simulink model "lab07_Arduino"  (R2022b)
settings: Solver=FixedStepAuto  StartTime=0.0  StopTime=inf  RelTol=1e-3
libraries: arduinolib x4, simulink x3
(part 2 of 2)

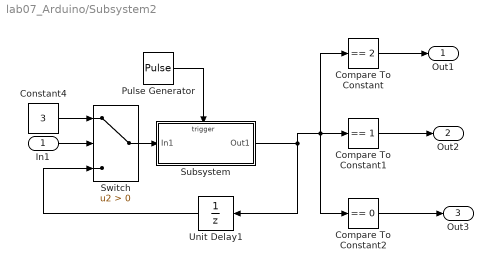
== system lab07_Arduino/Subsystem2 ==
  In1 : Inport
  Compare To Constant : simulink/Logic and Bit Operations/Compare To Constant  relop===  const=2  OutDataTypeStr=boolean
  Compare To Constant1 : simulink/Logic and Bit Operations/Compare To Constant  relop===  const=1  OutDataTypeStr=boolean
  Compare To Constant2 : simulink/Logic and Bit Operations/Compare To Constant  relop===  const=0  OutDataTypeStr=boolean
  Constant4 : Constant  Value=3
  Pulse Generator : DiscretePulseGenerator  PulseType=Time based  Period=5
  Subsystem : Subsystem
  Switch : Switch  Criteria=u2 > Threshold  SaturateOnIntegerOverflow=off  InputSameDT=off
  Unit Delay1 : UnitDelay  SampleTime=-1  HasFrameUpgradeWarning=on
  Out1 : Outport
  Out2 : Outport  Port=2
  Out3 : Outport  Port=3
  wires:
  Compare To Constant/1 -> Out1/1
  Compare To Constant1/1 -> Out2/1
  Compare To Constant2/1 -> Out3/1
  Constant4/1 -> Switch/1
  Unit Delay1/1 -> Switch/3
  In1/1 -> Switch/2
  Subsystem/1(Out1) -> Compare To Constant1/1, Compare To Constant2/1, Compare To Constant/1, Unit Delay1/1
  Switch/1 -> Subsystem/1(In1)
  Pulse Generator/1 -> Subsystem/Trigger

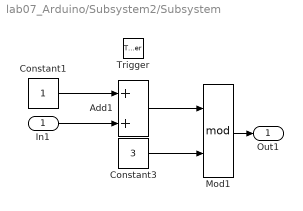
== system lab07_Arduino/Subsystem2/Subsystem ==
  In1 : Inport
  Trigger : TriggerPort  TriggerType=falling  VariantControl=(inherit)
  Add1 : Sum
  Constant1 : Constant
  Constant3 : Constant  Value=3
  Mod1 : Math  Operator=mod
  Out1 : Outport
  wires:
  Constant1/1 -> Add1/1
  Constant3/1 -> Mod1/2
  Add1/1 -> Mod1/1
  In1/1 -> Add1/2
  Mod1/1 -> Out1/1
